simulink model "sim2"  (R2023b)
settings: Solver=VariableStepAuto  StartTime=0.0  StopTime=0.4  RelTol=1e-3
settings Model: Creator=denismatveev  LastModifiedBy=denismatveev

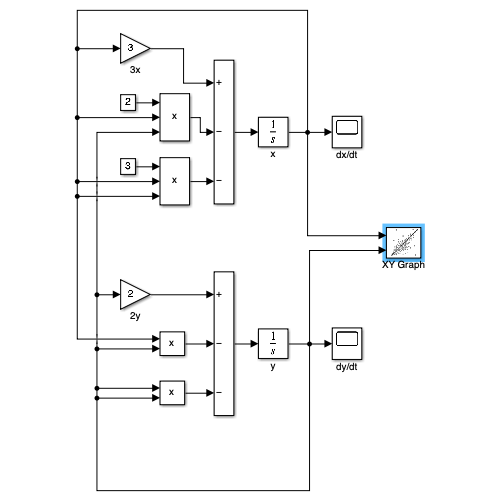
[thumbnail: Simulink's stored preview of the top-level diagram]
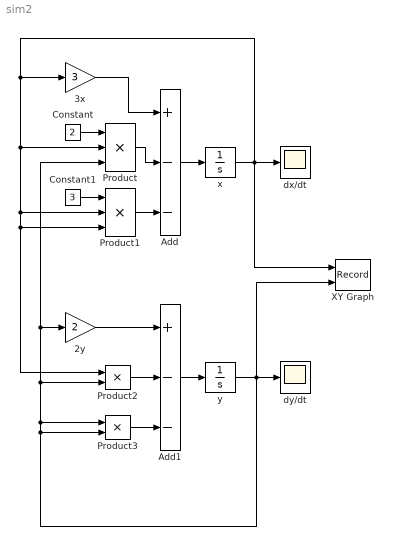
== system sim2 ==
  2y : Gain  Gain=2
  3x : Gain  Gain=3
  Add : Sum  Inputs=+--
  Add1 : Sum  Inputs=+--
  Constant : Constant  Value=2
  Constant1 : Constant  Value=3
  Product : Product  Inputs=3
  Product1 : Product  Inputs=3
  Product2 : Product
  Product3 : Product
  XY Graph : Record  FileSettingsInternal="{\"entries\":[{\"content\":{\"excelSettings\":{\"content\":{},\"type\":\"Streamout.ExcelSettings\"}},\"type\":\"Streamout.FileSettingStorage\",\"uuid\":\"\"}],\"packageUris\":[\"http:\\/\\/schema.mathworks.com\\/mf0\\/streamout_blocks\\/R2020a\"],\"version\":\"1.0\"}"  Layout=[1 1]  SignalsInternal="{\"entries\":[{\"content\":{\"signals\":[{\"content\":{\"blockPath\":[],\"dimensions\":[1],\"domain\":\"\",\"lineColor\":\"#a2142f\",\"plots\":[1],\"port\":1,\"sid\":[\"\"],\"signalID\":1805,\"signalName\":\"x\"},\"type\":\"RecordBlkView.Signal\",\"uuid\":\"\"},{\"content\":{\"blockPath\":[],\"dimensions\":[1],\"domain\":\"\",\"lineColor\":\"#139fff\",\"plots\":[1],\"port\":2,\"sid\":[\"\"],\"signalID\":1809,\"signalName\":\"y\"},\"type\":\"RecordBlkView.Signal\",\"uuid\":\"\"}]},\"type\":\"RecordBlkView.InputSignals\",\"uuid\":\"\"}],\"packageUris\":[\"http:\\/\\/schema.mathworks.com\\/mf0\\/streamout_blocks\\/R2020a\"],\"version\":\"1.0\"}"  VisualizationBindings="{\"xyplotplugin\":{\"info\":[{\"series\":[{\"bindingParametersList\":[{\"parameter\":\"X-Axis\",\"signalID\":1805,\"signalName\":\"x\"},{\"parameter\":\"Y-Axis\",\"signalID\":1809,\"signalName\":\"y\"}],\"seriesID\":31276}],\"subplotID\":1}]}}"  CompatibilityTag=XY
  dx/dt : Scope
  dy/dt : Scope
  x : Integrator  InitialCondition=-0.3
  y : Integrator  InitialCondition=-0.3
  wires:
  y/1 -> XY Graph/2, Product2/2, Product/3, 2y/1, Product3/1, Product3/2, dy/dt/1
  x/1 -> XY Graph/1, 3x/1, Product/2, Product1/2, Product2/1, Product1/3, dx/dt/1
  Add/1 -> x/1
  3x/1 -> Add/1
  Product/1 -> Add/2
  Constant/1 -> Product/1
  Product1/1 -> Add/3
  Constant1/1 -> Product1/1
  Add1/1 -> y/1
  2y/1 -> Add1/1
  Product2/1 -> Add1/2
  Product3/1 -> Add1/3
